simulink model "Loops6"  (Simulink 6.0)
settings: Solver=ode45  StartTime=0.0  StopTime=10.0  RelTol=1e-3
settings Model: Creator=scaife  LastModifiedBy=scaife  ExtModeAutoUpdateStatusClock=off
settings DataIOCC: SignalLoggingName=sigsOut
settings DebuggingCC: SolverPrmCheckMsg=none
settings HardwareCC: TargetUnknown=on
settings GRTTargetCC: ModelReferenceCompliant=off  MatFileLogging=off

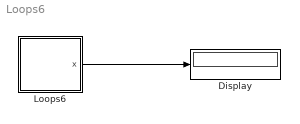
== system Loops6 ==
  Display : Display
  Loops6 : Stateflow chart
  wires:
  Loops6/1(x) -> Display/1

== stateflow chart Loops6 ==
  state A
  state B
  A -> (junction 5) : {x=0;}
  (junction 6) -> B
  (default) -> A
  (junction 7) -> B
  (junction 5) -> (junction 6) : [y]{y=!y;}
  (junction 5) -> (junction 7) : [!y]{y=!y;}
  (junction 7) -> (junction 5) : [x<2]{x++;}
  (junction 6) -> (junction 5) : [x<4]{x++;}
  data: x output int32; y local boolean
